simulink model "combinedTxRx_16bit"  (R2017a)
settings: Solver=FixedStepDiscrete  StartTime=0.0  StopTime=10.0  RelTol=1e-3
InitFcn:
  | numHeaderBits = 16;
  | %numPreambleBits = 250;
  | AGCBarkerSymbols = 160+28;
  | EQTrainingSymbols = 250;
  | CRCGeneratorLag = 34; % CRCLen + 2
  | 
  | %% AGC Preamble
  | B13bipolar = [0 0 0 0 0 2 2 0 0 2 0 2];
  | rep = [B13bipolar, B13bipolar(1:4)];
  | AGCBarker = repmat(rep,1,10);
  | % Second preamble part
  | B11bipolar = [0 0 0 2 2 2 0 2  2 0 2];
  | TimingBarker = [B11bipolar,B11bipolar,B11bipolar,B11bipolar(1:6)];
  | PreambleBarkersInts = [AGCBarker, TimingBarker];
  | % Convert integer into their bit representation
  | PreambleBarkersBits = zeros(1,length(PreambleBarkersInts)*2);
  | PreambleBarkersBits(1:2:end) = (PreambleBarkersInts==2);
  | 
  | % Constants
  | % First preamble part
  | B13bipolar = [0 0 0 0 0 2 2 0 0 2 0 2];
  | rep = [B13bipolar, B13bipolar(1:4)];
  | AGCBarker = repmat(rep,1,10);
  | % Second preamble part
  | B11bipolar = [0 0 0 2 2 2 0 2  2 0 2];
  | TimingBarker = [B11bipolar,B11bipolar,B11bipolar(1:6)];
  | PreambleBarkersInts = [AGCBarker, TimingBarker];
  | % Convert integer into their bit representation
  | PreambleBarkersBits = false(1,length(PreambleBarkersInts)*2);
  | PreambleBarkersBits(1:2:end) = logical(PreambleBarkersInts==2);
  | pLen = uint16(length(PreambleBarkersBits));
  | 
  | 
  | %%%%%%%%%%%%%%%%%%%%%%%%%%
  | %% RX
  | %%%%%%%%%%%%%%%%%%%%%%%%%%
  | 
  | barker = comm.BarkerCode('SamplesPerFrame', 28, 'Length', 11);
  | seq = barker()+1;
  | M = 4;
  | hPSKModTrain   = comm.PSKModulator(M, ...
  |     'PhaseOffset',pi/4, ...
  |     'SymbolMapping','Binary');
  | xPreambleSeq = hPSKModTrain(seq);
  | 
  | 
  | %%%%%%%%%%%%
  | 
  | % AGC Preamble
  | reps = 5;
  | barker = comm.BarkerCode('SamplesPerFrame', 16, 'Length', 13);
  | seq = barker()+1;
  | %preamble = zeros(16*reps,1);
  | preambleFull = repmat(seq,reps,1);
  | rctFilt = comm.RaisedCosineTransmitFilter('FilterSpanInSymbols', 128,...
  | 'RolloffFactor',0.5,...
  | 'OutputSamplesPerSymbol',4);
  | preambleFullFilt = rctFilt(preambleFull);
  | 
  | %%%%%%%%%%%%
  | 
  | RadioSampleRate = 1e6;
  | %RadioSampleRate = 20e6;
  | RadioFrameLength = 1e5;
  | 
  | VibertiTracebackLength = 34+20;
  | numTrainingSamples = 250;
  | crc32Poly = [1 0 0 0 0 0 1 0 0 1 1 0 0 0 0 0 1 0 0 0 1 1 1 0 1 1 0 1 1 0 1 1 1];
  | crcDecodeLag = length(crc32Poly)-1+2;
  | 
  | %%%%%%%%%%%%
  | 
  | beta = 0.5;
  | span = 8;
  | sps = 4;
  | filterGain = 1;
  | coeff = rcosdesign(beta, span, sps, 'sqrt')*filterGain;
  | 
  | %%%%%%%%%%%%
  | 
  | samplesPerSymbol = 4;
  | maxPacketBits = 8*1500;
  | bItsPerSymbol = 2;
  | CodeRate = 2;
  | tailSymbols = 40;
  | maxPayloadSymbols = maxPacketBits*CodeRate/bItsPerSymbol+tailSymbols;
undefined symbols (not defined in the file or in its folder): j
libraries: simulink x22, dsphdlfiltering x20, hdlsllib x6, commseqgen3 x4, dspsigops x4, commdigbbndpm3 x3, commcrc2 x2, commcnvcod2 x2, dspstat3 x2, commsource2 x1, commutil2 x1, commfilt2 x1
(part 1 of 3)
settings Model: Creator=tcollins  LastModifiedBy=tcollins
settings OptimizationCC: BlockReduction=off  ConditionallyExecuteInputs=off  DefaultParameterBehavior=Inlined
settings DebuggingCC: AlgebraicLoopMsg=error  SingleTaskRateTransMsg=error
settings HardwareCC: ProdBitPerPointer=32  ProdBitPerSizeT=32  ProdBitPerPtrDiffT=32  ProdLargestAtomicFloat=None  ProdIntDivRoundTo=Undefined  ProdEndianess=Unspecified  ProdWordSize=32  ProdHWDeviceType=ASIC/FPGA->ASIC/FPGA  ProdEqTarget=off

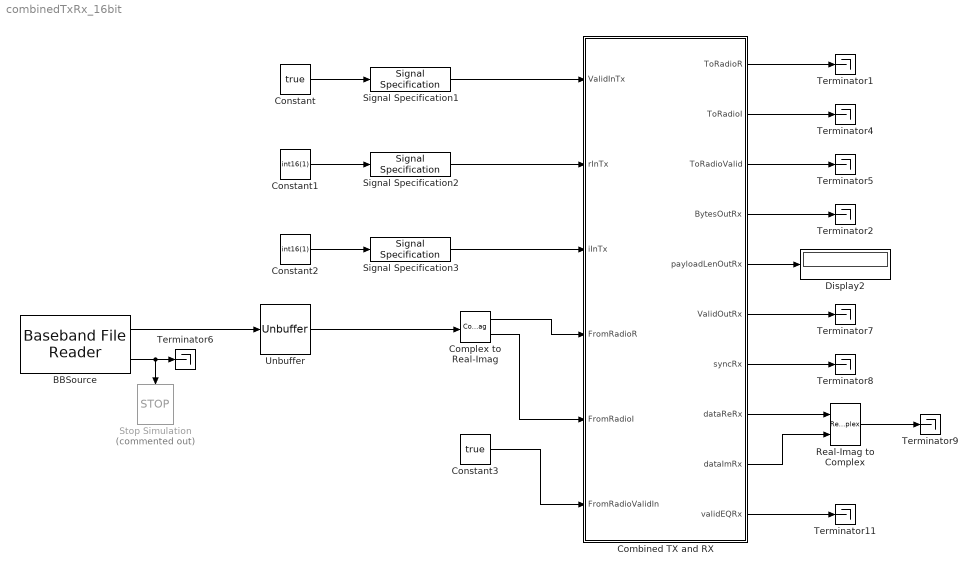
== system combinedTxRx_16bit ==
  BBSource : commsource2/Baseband File Reader  Filename=/home/tcollins/currentWork/modem-phy/FixedPoint/Pluto3.bb  InheritSampleTimeFromFile=off  SampleTime=100000/(RadioSampleRate)  SamplesPerFrame=100000  CyclicRepetition=off  FileEndOutputPort=on  SimulateUsing=Interpreted execution
      settings: SourceProductName=Communications System Toolbox  SourceProductBaseCode=CM
  Combined TX and RX : Subsystem  TreatAsAtomicUnit=on
  Complex to Real-Imag : ComplexToRealImag
  Constant : Constant  Value=true  SampleTime=-1
  Constant1 : Constant  Value=int16(1)  SampleTime=-1
  Constant2 : Constant  Value=int16(1)  SampleTime=-1
  Constant3 : Constant  Value=true  SampleTime=1/RadioSampleRate
  Display2 : Display
  Real-Imag to Complex : RealImagToComplex
  Signal Specification1 : SignalSpecification  OutDataTypeStr=boolean  SampleTime=1e-6
  Signal Specification2 : SignalSpecification  OutDataTypeStr=int16  SampleTime=1e-6
  Signal Specification3 : SignalSpecification  OutDataTypeStr=int16  SampleTime=1e-6
  Stop Simulation : Stop  Commented=on
  Terminator{1..2,4..9,11} (9 alike) : Terminator
  Unbuffer : Unbuffer
  wires:
  Constant1/1 -> Signal Specification2/1
  Constant2/1 -> Signal Specification3/1
  Constant/1 -> Signal Specification1/1
  Real-Imag to Complex/1 -> Terminator9/1
  BBSource/1 -> Unbuffer/1
  Unbuffer/1 -> Complex to Real-Imag/1
  BBSource/2 -> Stop Simulation/1, Terminator6/1
  Signal Specification1/1 -> Combined TX and RX/1(ValidInTx)
  Signal Specification2/1 -> Combined TX and RX/2(rInTx)
  Signal Specification3/1 -> Combined TX and RX/3(iInTx)
  Complex to Real-Imag/1 -> Combined TX and RX/4(FromRadioR)
  Complex to Real-Imag/2 -> Combined TX and RX/5(FromRadioI)
  Constant3/1 -> Combined TX and RX/6(FromRadioValidIn)
  Combined TX and RX/1(ToRadioR) -> Terminator1/1
  Combined TX and RX/2(ToRadioI) -> Terminator4/1
  Combined TX and RX/3(ToRadioValid) -> Terminator5/1
  Combined TX and RX/4(BytesOutRx) -> Terminator2/1
  Combined TX and RX/5(payloadLenOutRx) -> Display2/1
  Combined TX and RX/6(ValidOutRx) -> Terminator7/1
  Combined TX and RX/7(syncRx) -> Terminator8/1
  Combined TX and RX/8(dataReRx) -> Real-Imag to Complex/1
  Combined TX and RX/9(dataImRx) -> Real-Imag to Complex/2
  Combined TX and RX/10(validEQRx) -> Terminator11/1

== system combinedTxRx_16bit/Combined TX and RX ==
  ValidInTx : Inport
  rInTx : Inport  Port=2
  iInTx : Inport  Port=3
  FromRadioR : Inport  Port=4
  FromRadioI : Inport  Port=5
  FromRadioValidIn : Inport  Port=6
  Receiver HDL : Subsystem  TreatAsAtomicUnit=on
  Tx Under Test : Subsystem  TreatAsAtomicUnit=on
  ToRadioR : Outport
  ToRadioI : Outport  Port=2
  ToRadioValid : Outport  Port=3
  BytesOutRx : Outport  Port=4
  payloadLenOutRx : Outport  Port=5
  ValidOutRx : Outport  Port=6
  syncRx : Outport  Port=7
  dataReRx : Outport  Port=8
  dataImRx : Outport  Port=9
  validEQRx : Outport  Port=10
  wires:
  Receiver HDL/2(validOut) -> ValidOutRx/1
  Receiver HDL/6(dataIm) -> dataImRx/1
  Receiver HDL/3(sync) -> syncRx/1
  FromRadioI/1 -> Receiver HDL/2(Im)
  Receiver HDL/4(payloadLenOut) -> payloadLenOutRx/1
  Receiver HDL/7(validEQ) -> validEQRx/1
  Receiver HDL/5(dataRe) -> dataReRx/1
  FromRadioValidIn/1 -> Receiver HDL/3(Enable)
  FromRadioR/1 -> Receiver HDL/1(re)
  Receiver HDL/1(bytesOut) -> BytesOutRx/1
  rInTx/1 -> Tx Under Test/2("r ")
  Tx Under Test/2(Out2) -> ToRadioI/1
  Tx Under Test/3(Out3) -> ToRadioValid/1
  Tx Under Test/1(Out1) -> ToRadioR/1
  iInTx/1 -> Tx Under Test/3(i)
  ValidInTx/1 -> Tx Under Test/1(In1)

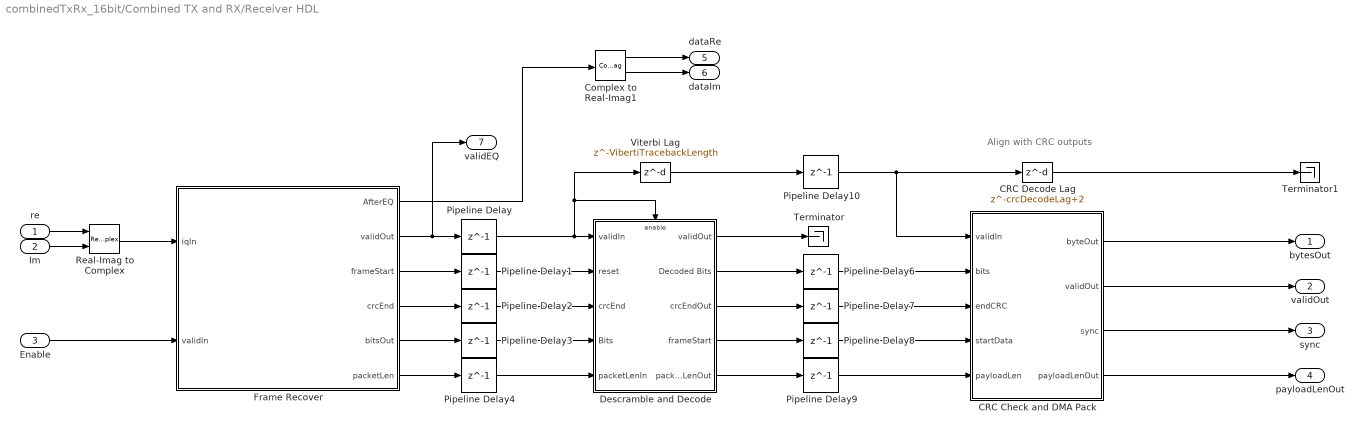
== system combinedTxRx_16bit/Combined TX and RX/Receiver HDL ==
  note: Align with CRC outputs
  re : Inport  OutDataTypeStr=int16
  Im : Inport  Port=2  OutDataTypeStr=int16
  Enable : Inport  Port=3
  CRC Check and DMA Pack : Subsystem
  CRC Decode Lag : Delay  DelayLength=crcDecodeLag+2
  Complex to Real-Imag1 : ComplexToRealImag
  Descramble and Decode : Subsystem  TreatAsAtomicUnit=on
  Frame Recover : Subsystem
  Pipeline Delay{,1..4,6..10} (10 alike) : Delay  DelayLength=1
  Real-Imag to Complex : RealImagToComplex
  Terminator : Terminator
  Terminator1 : Terminator
  Viterbi Lag : Delay  DelayLength=VibertiTracebackLength
  bytesOut : Outport
  validOut : Outport  Port=2
  sync : Outport  Port=3
  payloadLenOut : Outport  Port=4
  dataRe : Outport  Port=5
  dataIm : Outport  Port=6
  validEQ : Outport  Port=7
  wires:
  re/1 -> Real-Imag to Complex/1
  Im/1 -> Real-Imag to Complex/2
  Complex to Real-Imag1/2 -> dataIm/1
  Complex to Real-Imag1/1 -> dataRe/1
  Frame Recover/6(packetLen) -> Pipeline Delay4/1
  Frame Recover/2(validOut) -> validEQ/1, Pipeline Delay/1
  Real-Imag to Complex/1 -> Frame Recover/1(iqIn)
  Enable/1 -> Frame Recover/2(validIn)
  Frame Recover/1(AfterEQ) -> Complex to Real-Imag1/1
  Frame Recover/3(frameStart) -> Pipeline Delay1/1
  Frame Recover/4(crcEnd) -> Pipeline Delay2/1
  Frame Recover/5(bitsOut) -> Pipeline Delay3/1
  Descramble and Decode/3(crcEndOut) -> Pipeline Delay7/1
  Descramble and Decode/4(frameStart) -> Pipeline Delay8/1
  Descramble and Decode/5(packetLenOut) -> Pipeline Delay9/1
  CRC Check and DMA Pack/1(byteOut) -> bytesOut/1
  CRC Check and DMA Pack/2(validOut) -> validOut/1
  Pipeline Delay1/1 -> Descramble and Decode/2(reset)
  Pipeline Delay3/1 -> Descramble and Decode/4(Bits)
  Pipeline Delay4/1 -> Descramble and Decode/5(packetLenIn)
  Pipeline Delay8/1 -> CRC Check and DMA Pack/4(startData)
  Pipeline Delay6/1 -> CRC Check and DMA Pack/2(bits)
  Pipeline Delay9/1 -> CRC Check and DMA Pack/5(payloadLen)
  Pipeline Delay7/1 -> CRC Check and DMA Pack/3(endCRC)
  CRC Check and DMA Pack/3(sync) -> sync/1
  Pipeline Delay2/1 -> Descramble and Decode/3(crcEnd)
  Descramble and Decode/2(Decoded Bits) -> Pipeline Delay6/1
  Pipeline Delay10/1 -> CRC Check and DMA Pack/1(validIn), CRC Decode Lag/1
  CRC Check and DMA Pack/4(payloadLenOut) -> payloadLenOut/1
  Pipeline Delay/1 -> Descramble and Decode/Enable, Viterbi Lag/1, Descramble and Decode/1(validIn)
  Descramble and Decode/1(validOut) -> Terminator/1
  Viterbi Lag/1 -> Pipeline Delay10/1
  CRC Decode Lag/1 -> Terminator1/1

== system combinedTxRx_16bit/Combined TX and RX/Tx Under Test ==
  note: Keep On
  In1 : Inport
  "r " : Inport  Port=2
  i : Inport  Port=3
  DMA Model Driver : MATLAB Function  TreatAsAtomicUnit=on
  Data Type Conversion : DataTypeConversion  OutDataTypeStr=uint16
  Delay : Delay  DelayLength=1
  Downsample1 : DownSample  N=4  RateOptions=Allow multirate processing
  Downsample2 : DownSample  N=4  RateOptions=Allow multirate processing
  Logical Operator : Logic  Operator=OR  AllPortsSameDT=off  OutDataTypeStr=boolean
  Logical Operator1 : Logic  Operator=NOT  AllPortsSameDT=off  OutDataTypeStr=boolean
  Terminator : Terminator
  Terminator1 : Terminator
  Transmitter HDL : Subsystem  TreatAsAtomicUnit=on
  Upsample : dspsigops/Upsample  N=4  phase=0  RateOptions=Allow multirate processing  ic=0  mode=Unused parameter value
  Upsample1 : dspsigops/Upsample  N=4  phase=0  RateOptions=Allow multirate processing  ic=0  mode=Unused parameter value
  Out1 : Outport
  Out2 : Outport  Port=2
  Out3 : Outport  Port=3
  wires:
  Transmitter HDL/4(Need Data) -> Downsample1/1
  Transmitter HDL/2(imag) -> Out2/1
  Transmitter HDL/1(real) -> Out1/1
  Transmitter HDL/3(validOut) -> Out3/1
  DMA Model Driver/1(payload) -> Data Type Conversion/1
  Delay/1 -> DMA Model Driver/2(enable)
  In1/1 -> Downsample2/1
  Data Type Conversion/1 -> Upsample/1
  DMA Model Driver/2(valid) -> Upsample1/1
  "r "/1 -> Terminator/1
  i/1 -> Terminator1/1
  Upsample/1 -> Transmitter HDL/1(bytesIn)
  Upsample1/1 -> Transmitter HDL/2(validIn)
  Downsample1/1 -> Delay/1
  Logical Operator/1 -> DMA Model Driver/1(driver)
  Logical Operator1/1 -> Logical Operator/2
  Downsample2/1 -> Logical Operator1/1, Logical Operator/1

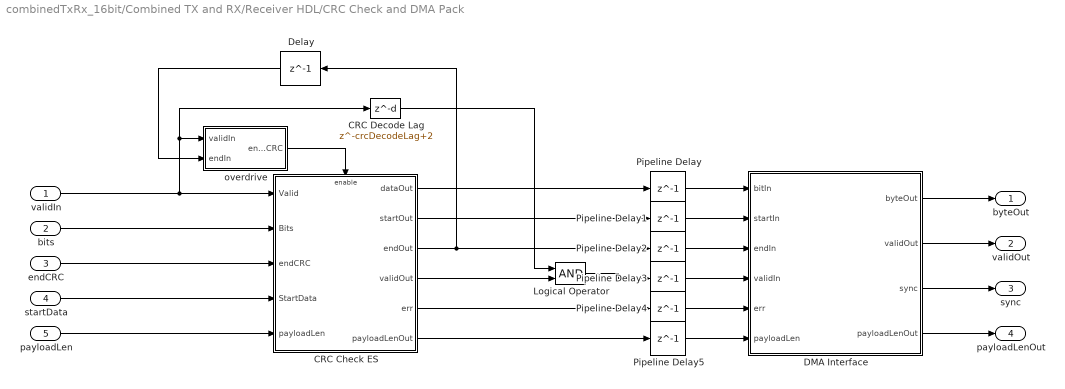
== system combinedTxRx_16bit/Combined TX and RX/Receiver HDL/CRC Check and DMA Pack ==
  validIn : Inport
  bits : Inport  Port=2
  endCRC : Inport  Port=3
  startData : Inport  Port=4
  payloadLen : Inport  Port=5
  CRC Check ES : Subsystem
  CRC Decode Lag : Delay  DelayLength=crcDecodeLag+2
  DMA Interface : Subsystem
  Delay : Delay  DelayLength=1
  Logical Operator : Logic  AllPortsSameDT=off  OutDataTypeStr=boolean
  Pipeline Delay{,1..5} (6 alike) : Delay  DelayLength=1
  overdrive : MATLAB Function  TreatAsAtomicUnit=on
  byteOut : Outport
  validOut : Outport  Port=2
  sync : Outport  Port=3
  payloadLenOut : Outport  Port=4
  wires:
  DMA Interface/2(validOut) -> validOut/1
  CRC Check ES/3(endOut) -> Delay/1, Pipeline Delay2/1
  DMA Interface/1(byteOut) -> byteOut/1
  CRC Check ES/2(startOut) -> Pipeline Delay1/1
  CRC Check ES/1(dataOut) -> Pipeline Delay/1
  CRC Check ES/5(err) -> Pipeline Delay4/1
  bits/1 -> CRC Check ES/2(Bits)
  DMA Interface/3(sync) -> sync/1
  payloadLen/1 -> CRC Check ES/5(payloadLen)
  startData/1 -> CRC Check ES/4(StartData)
  CRC Check ES/6(payloadLenOut) -> Pipeline Delay5/1
  endCRC/1 -> CRC Check ES/3(endCRC)
  Pipeline Delay/1 -> DMA Interface/1(bitIn)
  Pipeline Delay1/1 -> DMA Interface/2(startIn)
  Pipeline Delay2/1 -> DMA Interface/3(endIn)
  Pipeline Delay3/1 -> DMA Interface/4(validIn)
  Pipeline Delay4/1 -> DMA Interface/5(err)
  Pipeline Delay5/1 -> DMA Interface/6(payloadLen)
  CRC Decode Lag/1 -> Logical Operator/1
  CRC Check ES/4(validOut) -> Logical Operator/2
  validIn/1 -> CRC Check ES/1(Valid), CRC Decode Lag/1, overdrive/1(validIn)
  Delay/1 -> overdrive/2(endIn)
  DMA Interface/4(payloadLenOut) -> payloadLenOut/1
  Logical Operator/1 -> Pipeline Delay3/1
  overdrive/1(enableCRC) -> CRC Check ES/Enable

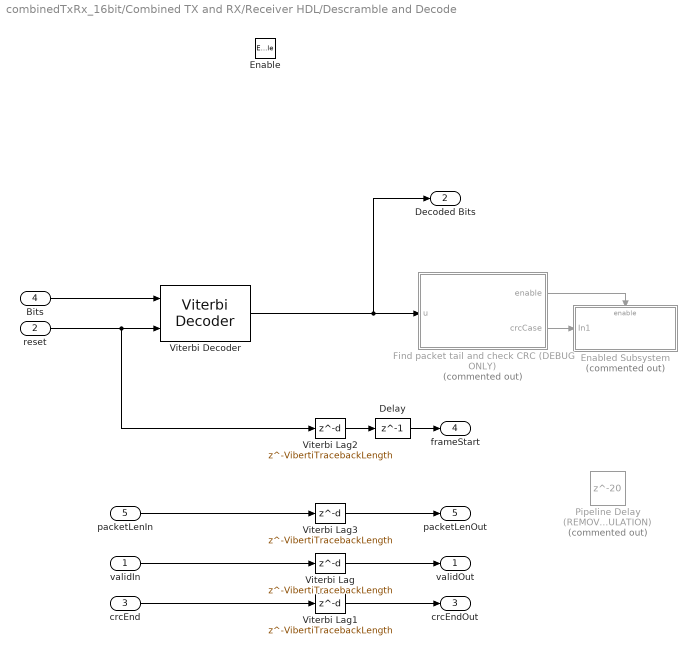
== system combinedTxRx_16bit/Combined TX and RX/Receiver HDL/Descramble and Decode ==
  validIn : Inport
  reset : Inport  Port=2
  crcEnd : Inport  Port=3
  Bits : Inport  Port=4
  packetLenIn : Inport  Port=5
  Enable : EnablePort
  Delay : Delay  DelayLength=1
  Enabled Subsystem : Subsystem  Commented=on  TreatAsAtomicUnit=on
  Find packet tail and check CRC (DEBUG ONLY) : MATLAB Function  Commented=on  TreatAsAtomicUnit=on
  "Pipeline Delay (REMOVE BEFORE SYNTH, ONLY FOR SIMULATION)" : Delay  Commented=on  DelayLength=20
  Viterbi Decoder : commcnvcod2/Viterbi Decoder  trellis=poly2trellis(7, [171 133])  isPunctured=off  punctureVector=[1; 1; 0; 1; 0; 1]  erasures=off  dectype=Hard decision  nsdecb=4  runSigValErrCheck=off  tbdepth=VibertiTracebackLength-20  opmode=Continuous  reset=on  delayedResetAction=on  smWordLength=16  outDataType=boolean
      settings: SourceProductName=Communications System Toolbox  SourceProductBaseCode=CM
  Viterbi Lag{,1..3} (4 alike) : Delay  DelayLength=VibertiTracebackLength
  validOut : Outport  InitialOutput=0
  Decoded Bits : Outport  Port=2  InitialOutput=0
  crcEndOut : Outport  Port=3  InitialOutput=0
  frameStart : Outport  Port=4  InitialOutput=0
  packetLenOut : Outport  Port=5  InitialOutput=0
  wires:
  reset/1 -> Viterbi Lag2/1, Viterbi Decoder/2
  Find packet tail and check CRC (DEBUG ONLY)/1(enable) -> Enabled Subsystem/Enable
  Find packet tail and check CRC (DEBUG ONLY)/2(crcCase) -> Enabled Subsystem/1(In1)
  Bits/1 -> Viterbi Decoder/1
  validIn/1 -> Viterbi Lag/1
  Viterbi Lag3/1 -> packetLenOut/1
  Viterbi Lag2/1 -> Delay/1
  Viterbi Lag1/1 -> crcEndOut/1
  Viterbi Lag/1 -> validOut/1
  packetLenIn/1 -> Viterbi Lag3/1
  crcEnd/1 -> Viterbi Lag1/1
  Delay/1 -> frameStart/1
  Viterbi Decoder/1 -> Decoded Bits/1, Find packet tail and check CRC (DEBUG ONLY)/1(u)

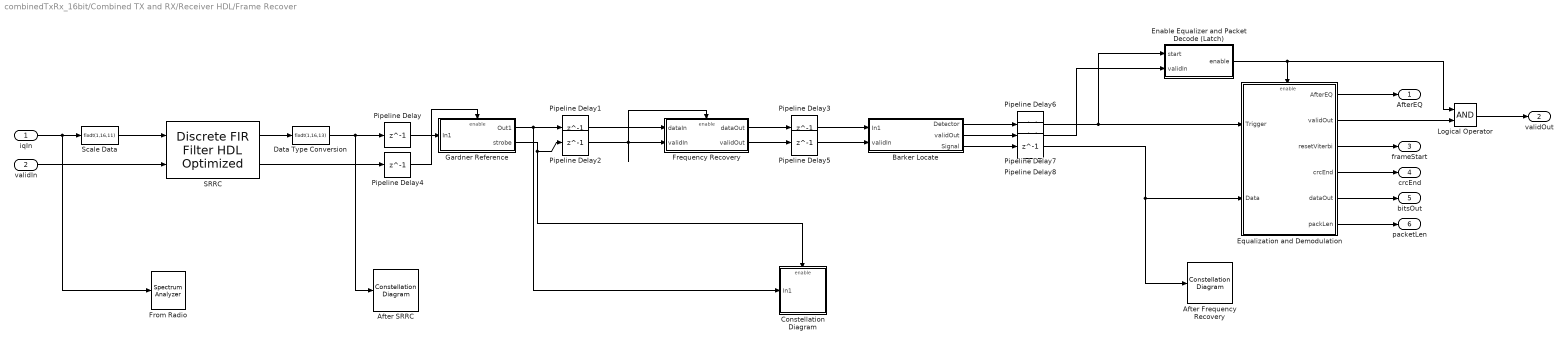
== system combinedTxRx_16bit/Combined TX and RX/Receiver HDL/Frame Recover ==
  iqIn : Inport
  validIn : Inport  Port=2
  After Frequency Recovery : ConstellationDiagram
  After SRRC : ConstellationDiagram
  Barker Locate : Subsystem  mask{Threshold=1}
  Constellation Diagram : Subsystem
  Data Type Conversion : DataTypeConversion  OutDataTypeStr=fixdt(1,16,13)
  Enable Equalizer and Packet Decode (Latch) : MATLAB Function  TreatAsAtomicUnit=on
  Equalization and Demodulation : Subsystem
  Frequency Recovery : Subsystem
  From Radio : SpectrumAnalyzer
  Gardner Reference : Subsystem
  Logical Operator : Logic  AllPortsSameDT=off  OutDataTypeStr=boolean
  Pipeline Delay{,1..8} (9 alike) : Delay  DelayLength=1
  SRRC : dsphdlfiltering/Discrete FIR Filter HDL Optimized  Numerator=coeff  Sharing=off  SharingFactor=2  SimulateUsing=Code generation  roundingMode=Floor  overflowMode=on  CoefficientsDataTypeStr=Inherit: Same word length as input  CoefficientsMin=[]  CoefficientsMax=[]  OutputDataTypeStr=fixdt(1,16,11)  OutputMin=[]  OutputMax=[]  ValidInPort=on  ReadyPort=off
      settings: SourceProductName=DSP System Toolbox  SourceProductBaseCode=DS
  Scale Data : DataTypeConversion  OutDataTypeStr=fixdt(1,16,11)  ConvertRealWorld=Stored Integer (SI)  SaturateOnIntegerOverflow=on
  AfterEQ : Outport
  validOut : Outport  Port=2
  frameStart : Outport  Port=3
  crcEnd : Outport  Port=4
  bitsOut : Outport  Port=5
  packetLen : Outport  Port=6
  wires:
  Equalization and Demodulation/3(resetViterbi) -> frameStart/1
  Barker Locate/2(validOut) -> Pipeline Delay7/1
  Equalization and Demodulation/4(crcEnd) -> crcEnd/1
  Frequency Recovery/2(validOut) -> Pipeline Delay5/1
  Enable Equalizer and Packet Decode (Latch)/1(enable) -> Logical Operator/1, Equalization and Demodulation/Enable
  Equalization and Demodulation/5(dataOut) -> bitsOut/1
  SRRC/2 -> Pipeline Delay4/1
  SRRC/1 -> Data Type Conversion/1
  iqIn/1 -> From Radio/1, Scale Data/1
  validIn/1 -> SRRC/2
  Barker Locate/3(Signal) -> Pipeline Delay8/1
  Frequency Recovery/1(dataOut) -> Pipeline Delay3/1
  Equalization and Demodulation/2(validOut) -> Logical Operator/2
  Scale Data/1 -> SRRC/1
  Equalization and Demodulation/6(packLen) -> packetLen/1
  Barker Locate/1(Detector) -> Pipeline Delay6/1
  Equalization and Demodulation/1(AfterEQ) -> AfterEQ/1
  Pipeline Delay1/1 -> Frequency Recovery/1(dataIn)
  Pipeline Delay2/1 -> Frequency Recovery/Enable, Frequency Recovery/2(validIn)
  Pipeline Delay3/1 -> Barker Locate/1(In1)
  Pipeline Delay5/1 -> Barker Locate/2(validIn)
  Pipeline Delay6/1 -> Enable Equalizer and Packet Decode (Latch)/1(start), Equalization and Demodulation/1(Trigger)
  Pipeline Delay7/1 -> Enable Equalizer and Packet Decode (Latch)/2(validIn)
  Pipeline Delay8/1 -> Equalization and Demodulation/2(Data), After Frequency Recovery/1
  Logical Operator/1 -> validOut/1
  Data Type Conversion/1 -> After SRRC/1, Pipeline Delay/1
  Pipeline Delay/1 -> Gardner Reference/1(In1)
  Gardner Reference/2(strobe) -> Pipeline Delay2/1, Constellation Diagram/Enable
  Gardner Reference/1(Out1) -> Constellation Diagram/1(In1), Pipeline Delay1/1
  Pipeline Delay4/1 -> Gardner Reference/Enable

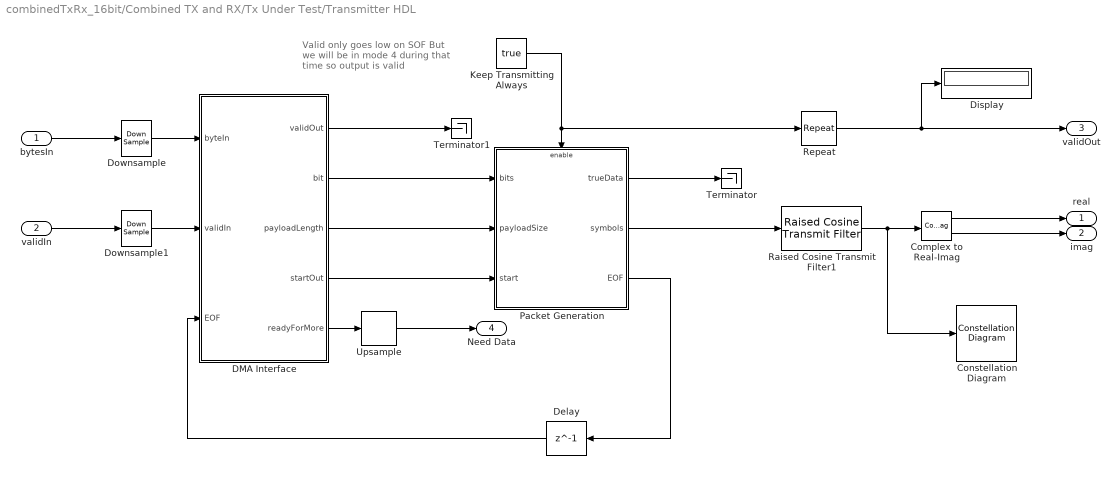
== system combinedTxRx_16bit/Combined TX and RX/Tx Under Test/Transmitter HDL ==
  note: Valid only goes low on SOF
      | But we will be in mode 4 during
      | that time so output is valid
  bytesIn : Inport
  validIn : Inport  Port=2
  Complex to Real-Imag : ComplexToRealImag
  Constellation Diagram : ConstellationDiagram
  DMA Interface : Subsystem
  Delay : Delay  DelayLength=1
  Display : Display
  Downsample : DownSample  N=4  RateOptions=Allow multirate processing
  Downsample1 : DownSample  N=4  RateOptions=Allow multirate processing
  Keep Transmitting Always : Constant  Value=true  SampleTime=-1
  Packet Generation : Subsystem
  Raised Cosine Transmit Filter1 : commfilt2/Raised Cosine Transmit Filter  filtType=Square root  R=0.5  filtSpan=8  N=4  filterGain=1  RateOptions=Allow multirate processing  framing=Mute  checkCoeff=off  variableName=rcTxFilt1  checkGain=Normalized  sampMode=Mute  saveAsFlag=0  currentFiltSpan=8  D=(8)/2  launchFVT=on  roundingMode=Floor  overflowMode=off  coeffDataTypeStr=Inherit: Same word length as input  coeffMin=[]  coeffMax=[]  coeffLastDataTypeStr=Inherit: Same word length as input  outputMode=Binary point scaling  outputWordLength=16  outputFracLength=14  outputDataTypeStr=fixdt(1,16,14)  outputMin=[]  outputMax=[]  outputLastDataTypeStr=fixdt(1,16,14)
  Repeat : dspsigops/Repeat  N=4  InputProcessing=Columns as channels (frame based)  RateOptions=Allow multirate processing  ic=0  mode=Unused parameter value
      settings: SourceProductName=DSP System Toolbox
  Terminator : Terminator
  Terminator1 : Terminator
  Upsample : dspsigops/Upsample  N=4  phase=0  RateOptions=Allow multirate processing  ic=0  mode=Unused parameter value
  real : Outport
  imag : Outport  Port=2
  validOut : Outport  Port=3
  Need Data : Outport  Port=4
  wires:
  Raised Cosine Transmit Filter1/1 -> Constellation Diagram/1, Complex to Real-Imag/1
  Complex to Real-Imag/1 -> real/1
  Complex to Real-Imag/2 -> imag/1
  DMA Interface/2(bit) -> Packet Generation/1(bits)
  DMA Interface/3(payloadLength) -> Packet Generation/2(payloadSize)
  DMA Interface/4(startOut) -> Packet Generation/3(start)
  Packet Generation/2(symbols) -> Raised Cosine Transmit Filter1/1
  DMA Interface/5(readyForMore) -> Upsample/1
  Repeat/1 -> validOut/1, Display/1
  Packet Generation/1(trueData) -> Terminator/1
  Packet Generation/3(EOF) -> Delay/1
  Delay/1 -> DMA Interface/3(EOF)
  bytesIn/1 -> Downsample/1
  validIn/1 -> Downsample1/1
  Upsample/1 -> Need Data/1
  Downsample/1 -> DMA Interface/1(byteIn)
  Downsample1/1 -> DMA Interface/2(validIn)
  DMA Interface/1(validOut) -> Terminator1/1
  Keep Transmitting Always/1 -> Packet Generation/Enable, Repeat/1

== system combinedTxRx_16bit/Combined TX and RX/Receiver HDL/CRC Check and DMA Pack/CRC Check ES ==
  note: NOTE:
      | 	The Valid signal must be latched during a packet, which is
      | 	a bug.  Therefore we must use the CRC block in an enabled
      | 	subsystem
  note: CRC Requires
      | Always High
      | Valid Signal During
      | Packet
  Valid : Inport
  Bits : Inport  Port=2
  endCRC : Inport  Port=3
  StartData : Inport  Port=4
  payloadLen : Inport  Port=5
  Enable : EnablePort
  CRC Decode Lag : Delay  DelayLength=crcDecodeLag
  Check CRC Result (DEBUG) : MATLAB Function  TreatAsAtomicUnit=on
  Convert To fi : DataTypeConversion  OutDataTypeStr=fixdt(0,1,0)  SaturateOnIntegerOverflow=on
  Debug CRC input : MATLAB Function  Commented=on  TreatAsAtomicUnit=on
  General CRC Syndrom Detector HDL Optimized : commcrc2/General CRC Syndrome Detector HDL Optimized  Polynomial=crc32Poly  InitialState=0  DirectMethod=off  ReflectInput=off  ReflectCRCChecksum=off  FinalXORValue=0  SimulateUsing=Code generation
      settings: SourceProductName=Communications System Toolbox  SourceProductBaseCode=CM
  dataOut : Outport  InitialOutput=0
  startOut : Outport  Port=2  InitialOutput=0
  endOut : Outport  Port=3  InitialOutput=0
  validOut : Outport  Port=4  InitialOutput=0
  err : Outport  Port=5  InitialOutput=0
  payloadLenOut : Outport  Port=6  InitialOutput=0
  wires:
  Bits/1 -> Convert To fi/1, Debug CRC input/1(u)
  General CRC Syndrom Detector HDL Optimized/1 -> Check CRC Result (DEBUG)/1(bits), dataOut/1
  General CRC Syndrom Detector HDL Optimized/3 -> Check CRC Result (DEBUG)/3(done), endOut/1
  General CRC Syndrom Detector HDL Optimized/4 -> Check CRC Result (DEBUG)/4(valid), validOut/1
  General CRC Syndrom Detector HDL Optimized/5 -> Check CRC Result (DEBUG)/5(err), err/1
  General CRC Syndrom Detector HDL Optimized/2 -> Check CRC Result (DEBUG)/2(start), startOut/1
  Convert To fi/1 -> General CRC Syndrom Detector HDL Optimized/1
  payloadLen/1 -> CRC Decode Lag/1
  CRC Decode Lag/1 -> payloadLenOut/1
  StartData/1 -> Debug CRC input/4(startFlag), General CRC Syndrom Detector HDL Optimized/2
  endCRC/1 -> Debug CRC input/3(endFlag), General CRC Syndrom Detector HDL Optimized/3
  Valid/1 -> Debug CRC input/2(enable), General CRC Syndrom Detector HDL Optimized/4

== system combinedTxRx_16bit/Combined TX and RX/Receiver HDL/CRC Check and DMA Pack/DMA Interface ==
  bitIn : Inport
  startIn : Inport  Port=2
  endIn : Inport  Port=3
  validIn : Inport  Port=4
  err : Inport  Port=5
  payloadLen : Inport  Port=6
  Bit Packer : MATLAB Function  TreatAsAtomicUnit=on
  Convert Payload Length To Bytes : Subsystem
  Data Type Conversion : DataTypeConversion  OutDataTypeStr=boolean
  Delay : Delay  DelayLength=1
  Delay Error To Last Byte of Out : Delay  DelayLength=1
  Display : Display
  byteOut : Outport
  validOut : Outport  Port=2
  sync : Outport  Port=3
  payloadLenOut : Outport  Port=4
  wires:
  bitIn/1 -> Data Type Conversion/1
  Delay/1 -> Bit Packer/3(endIn)
  Delay Error To Last Byte of Out/1 -> Bit Packer/4(err)
  Bit Packer/2(validOut) -> validOut/1
  Bit Packer/3(startOut) -> sync/1
  Bit Packer/1(byteOut) -> Display/1, byteOut/1
  err/1 -> Delay Error To Last Byte of Out/1
  validIn/1 -> Bit Packer/5(validIn)
  endIn/1 -> Delay/1
  startIn/1 -> Bit Packer/2(startIn)
  Data Type Conversion/1 -> Bit Packer/1(bitIn)
  payloadLen/1 -> Convert Payload Length To Bytes/1(In1)
  Convert Payload Length To Bytes/1(Out1) -> payloadLenOut/1

== system combinedTxRx_16bit/Combined TX and RX/Receiver HDL/Descramble and Decode/Enabled Subsystem ==
  In1 : Inport
  Enable : EnablePort
  To Workspace : ToWorkspace  VariableName=crcConditions  SaveFormat=Structure  SampleTime=-1
  wires:
  In1/1 -> To Workspace/1

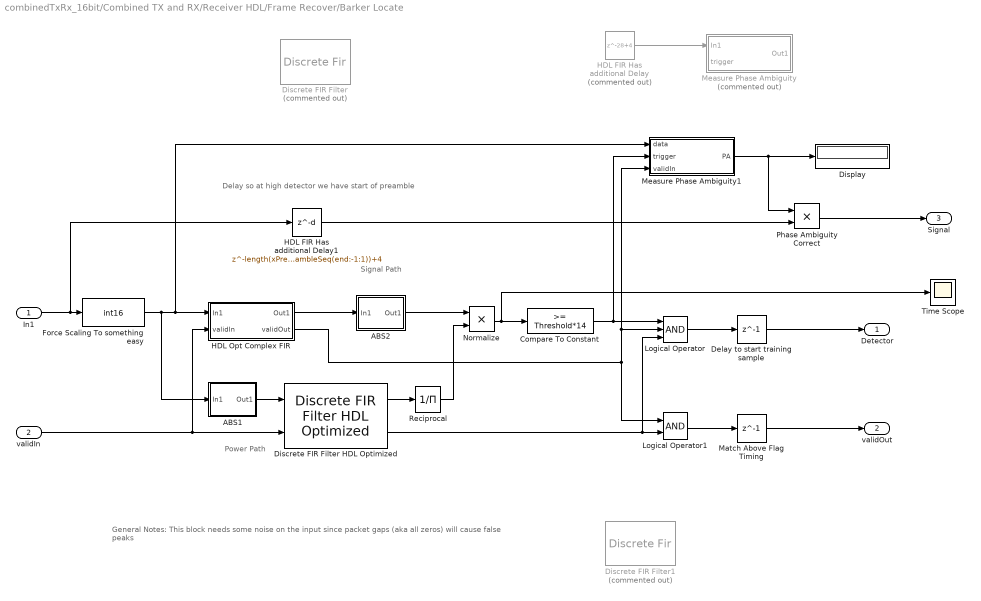
== system combinedTxRx_16bit/Combined TX and RX/Receiver HDL/Frame Recover/Barker Locate ==
  note: General Notes:
      | This block needs some noise on the input since packet gaps (aka all zeros) will cause false peaks
  note: Delay so at high detector we have start of preamble
  note: Power Path
  note: Signal Path
  In1 : Inport
  validIn : Inport  Port=2
  ABS1 : Subsystem
  ABS2 : Subsystem
  Compare To Constant : simulink/Logic and Bit Operations/Compare To Constant  relop=>=  const=Threshold*14  OutDataTypeStr=boolean
  "Delay to start training sample " : Delay  DelayLength=1
  Discrete FIR Filter : DiscreteFir  Commented=on  Coefficients=xPreambleSeq(end:-1:1).'  AccumDataTypeStr=Inherit: Same as product output  OutDataTypeStr=int16
  Discrete FIR Filter HDL Optimized : dsphdlfiltering/Discrete FIR Filter HDL Optimized  Numerator=ones(1,length(xPreambleSeq)*1)/1  Sharing=off  SharingFactor=2  SimulateUsing=Code generation  roundingMode=Floor  overflowMode=off  CoefficientsDataTypeStr=Inherit: Same word length as input  CoefficientsMin=[]  CoefficientsMax=[]  OutputDataTypeStr=fixdt(1,17,0)  OutputMin=[]  OutputMax=[]  ValidInPort=on  ReadyPort=off
      settings: SourceProductName=DSP System Toolbox  SourceProductBaseCode=DS
  Discrete FIR Filter1 : DiscreteFir  Commented=on  Coefficients=ones(1,length(xPreambleSeq)*1)/1  AccumDataTypeStr=Inherit: Same as product output  OutDataTypeStr=int16  SaturateOnIntegerOverflow=on
  Display : Display
  Force Scaling To something easy : DataTypeConversion  OutDataTypeStr=int16  SaturateOnIntegerOverflow=on
  HDL FIR Has additional Delay : Delay  Commented=on  DelayLength=28+4
  HDL FIR Has additional Delay1 : Delay  DelayLength=length(xPreambleSeq(end:-1:1))+4
  HDL Opt Complex FIR : Subsystem  mask{Taps=xPreambleSeq(end:-1:1).'}
  Logical Operator : Logic  Inputs=3  AllPortsSameDT=off  OutDataTypeStr=boolean
  Logical Operator1 : Logic  AllPortsSameDT=off  OutDataTypeStr=boolean
  Match Above Flag Timing : Delay  DelayLength=1
  Measure Phase Ambiguity : Subsystem  Commented=on
  Measure Phase Ambiguity1 : Subsystem
  Normalize : Product  Inputs=**  OutDataTypeStr=int16  RndMeth=Simplest  SaturateOnIntegerOverflow=on
  Phase Ambiguity Correct : Product  OutDataTypeStr=fixdt(1,16,14)
  Reciprocal : Product  Inputs=/  SaturateOnIntegerOverflow=on  RndMeth=Zero
  Time Scope : Scope
  Detector : Outport
  validOut : Outport  Port=2
  Signal : Outport  Port=3
  wires:
  HDL Opt Complex FIR/1(Out1) -> ABS2/1(In1)
  ABS2/1(Out1) -> Normalize/1
  "Delay to start training sample "/1 -> Detector/1
  Normalize/1 -> Time Scope/1, Compare To Constant/1
  In1/1 -> HDL FIR Has additional Delay1/1, Force Scaling To something easy/1
  ABS1/1(Out1) -> Discrete FIR Filter HDL Optimized/1
  Logical Operator/1 -> "Delay to start training sample "/1
  Logical Operator1/1 -> Match Above Flag Timing/1
  Measure Phase Ambiguity1/1(PA) -> Display/1, Phase Ambiguity Correct/1
  validIn/1 -> HDL Opt Complex FIR/2(validIn), Discrete FIR Filter HDL Optimized/2
  Discrete FIR Filter HDL Optimized/2 -> Logical Operator1/2, Logical Operator/3
  HDL Opt Complex FIR/2(validOut) -> Logical Operator1/1, Measure Phase Ambiguity1/3(validIn), Logical Operator/2
  Phase Ambiguity Correct/1 -> Signal/1
  HDL FIR Has additional Delay1/1 -> Phase Ambiguity Correct/2
  Force Scaling To something easy/1 -> ABS1/1(In1), HDL Opt Complex FIR/1(In1), Measure Phase Ambiguity1/1(data)
  Compare To Constant/1 -> Measure Phase Ambiguity1/2(trigger), Logical Operator/1
  HDL FIR Has additional Delay/1 -> Measure Phase Ambiguity/1(In1)
  Discrete FIR Filter HDL Optimized/1 -> Reciprocal/1
  Reciprocal/1 -> Normalize/2
  Match Above Flag Timing/1 -> validOut/1

== system combinedTxRx_16bit/Combined TX and RX/Receiver HDL/Frame Recover/Constellation Diagram ==
  In1 : Inport
  Enable : EnablePort
  After Timing Recovery : ConstellationDiagram
  wires:
  In1/1 -> After Timing Recovery/1

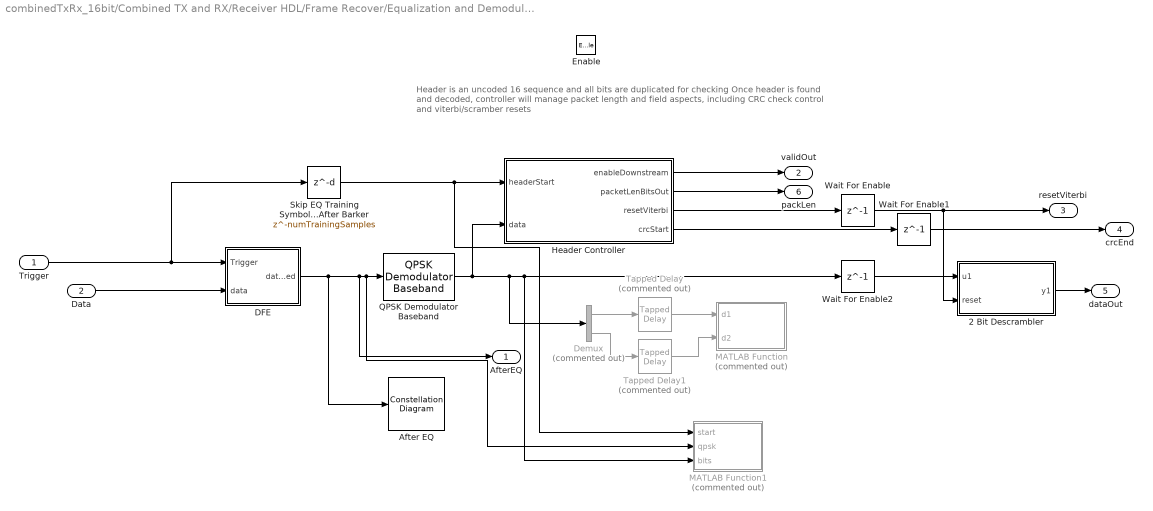
== system combinedTxRx_16bit/Combined TX and RX/Receiver HDL/Frame Recover/Equalization and Demodulation ==
  note: Header is an uncoded 16 sequence and all bits are duplicated for checking
      |
      | Once header is found and decoded, controller will manage packet length and field aspects,
      | including CRC check control and viterbi/scramber resets
  Trigger : Inport
  Data : Inport  Port=2
  Enable : EnablePort
  2 Bit Descrambler : Subsystem  mask{polynom=[1 1 0 1 0 1 0 1], initstate=[0 1 0 0 0 1 0]}
      mask prompts: polynom "Polynomial"; initstate "Inital State"
      mask Display: fprintf('HDL Descrambler')
  After EQ : ConstellationDiagram
  DFE : Subsystem
  Demux : Demux  Commented=on  Outputs=2
  Header Controller : MATLAB Function  TreatAsAtomicUnit=on
  MATLAB Function : MATLAB Function  Commented=on  TreatAsAtomicUnit=on
  MATLAB Function1 : MATLAB Function  Commented=on  TreatAsAtomicUnit=on
  QPSK Demodulator Baseband : commdigbbndpm3/QPSK Demodulator Baseband  OutType=Bit  DecType=Hard decision  VarSource=Dialog  Variance=1  Dec=Binary  Ph=pi/4  outDtype1=boolean  outDtype2=Inherit via internal rule  derotateFactorWordLen=16  derotateFactorDataTypeStr=Inherit: Same word length as input  derotateFactorLastDataTypeStr=Inherit: Same word length as input
  Skip EQ Training Symbols After Barker : Delay  DelayLength=numTrainingSamples
  Tapped Delay : simulink/Discrete/Tapped Delay  Commented=on  vinit=0.0  samptime=-1  NumDelays=16  DelayOrder=Oldest  includeCurrent=off
  Tapped Delay1 : simulink/Discrete/Tapped Delay  Commented=on  vinit=0.0  samptime=-1  NumDelays=16  DelayOrder=Oldest  includeCurrent=off
  Wait For Enable : Delay  DelayLength=1
  Wait For Enable1 : Delay  DelayLength=1
  Wait For Enable2 : Delay  DelayLength=1
  AfterEQ : Outport  InitialOutput=0
  validOut : Outport  Port=2  InitialOutput=0
  resetViterbi : Outport  Port=3  InitialOutput=0
  crcEnd : Outport  Port=4  InitialOutput=0
  dataOut : Outport  Port=5  InitialOutput=0
  packLen : Outport  Port=6  InitialOutput=0
  wires:
  Skip EQ Training Symbols After Barker/1 -> MATLAB Function1/1(start), Header Controller/1(headerStart)
  DFE/1(dataEQed) -> AfterEQ/1, MATLAB Function1/2(qpsk), QPSK Demodulator Baseband/1, After EQ/1
  QPSK Demodulator Baseband/1 -> Header Controller/2(data), Demux/1, MATLAB Function1/3(bits), Wait For Enable2/1
  Header Controller/1(enableDownstream) -> validOut/1
  Header Controller/4(crcStart) -> Wait For Enable1/1
  Header Controller/3(resetViterbi) -> Wait For Enable/1
  Header Controller/2(packetLenBitsOut) -> packLen/1
  Wait For Enable/1 -> 2 Bit Descrambler/2(reset), resetViterbi/1
  Wait For Enable1/1 -> crcEnd/1
  Wait For Enable2/1 -> 2 Bit Descrambler/1(u1)
  2 Bit Descrambler/1(y1) -> dataOut/1
  Demux/1 -> Tapped Delay/1
  Demux/2 -> Tapped Delay1/1
  Tapped Delay/1 -> MATLAB Function/1(d1)
  Tapped Delay1/1 -> MATLAB Function/2(d2)
  Trigger/1 -> DFE/1(Trigger), Skip EQ Training Symbols After Barker/1
  Data/1 -> DFE/2(data)

== system combinedTxRx_16bit/Combined TX and RX/Receiver HDL/Frame Recover/Frequency Recovery ==
  note: Decrease Loop bandwidth to reduce phase noise,
      | but worse pull-in range
      | -0.1 30kHz pull-in
      | -0.01 5kHz pull-in
  note: Max Phase Lock Delay= 1.3/(NormLoopBandwidth*SampleRate)
  note: Frequency Lock Delay = SampleRate*4*NormalizedPullInRange^2)/ (SampleRate*NormLoopBandwidth)^3;
  note: Pull in range (Hz) = 2*pi*sqrt(2)*DampingFactor*NormLoopBandwidth*SampleRate
  dataIn : Inport
  validIn : Inport  Port=2
  Enable : EnablePort
  Data Type Conversion : DataTypeConversion  Commented=on  OutDataTypeStr=fixdt(1,16,10)
  Delay : Delay  DelayLength=1
  Loop Filter : Subsystem  mask{BnTs=0.01, zeta=4*1/sqrt(2), N=1}
      mask prompts: BnTs "Normalized Loop Bandwidth"; zeta "Damping Factor"; N "Number of Samples/Symbol"
      mask init:
      | % See C.57 to C.61 in Michael Rice's "Digital Communications 
      | % - A Discrete-Time Approach" for details
      | 
      | %theta = BnTs/(zeta+0.25/zeta);  %0.0385
      | %d = 1 + 2*zeta*theta + theta*theta; %1.1938
      | %K1 = zeta*theta/d; %0.0805
      | %K2 = theta*theta/(d*2); %6.1958e-04
      | 
      | %%
      | DampingFactor = zeta;
      | samplesPerSymbol = N;
      | NormalizedLoopBandwidth = BnTs;
      | %
      | PhaseRecoveryLoopBandwidth = NormalizedLoopBandwidth*samplesPerSymbol;
      |  
      | PhaseRecoveryGain = samplesPerSymbol;
      |  
      | PhaseErrorDetectorGain = 1;
      | 
      | 
      | theta = PhaseRecoveryLoopBandwidth/...
      |     ((DampingFactor + 0.25/DampingFactor)*samplesPerSymbol);
      |  
      | d = 1 + 2*DampingFactor*theta + theta*theta;
      |  
      | % K1
      | K1 = (4*DampingFactor*theta/d)/...
      |     (PhaseErrorDetectorGain*PhaseRecoveryGain);
      | % K2
      | K2 = (4/samplesPerSymbol*theta*theta/d)/...
      |     (PhaseErrorDetectorGain*PhaseRecoveryGain);
      mask Display: disp('Loop Filter')
  PED : MATLAB Function  TreatAsAtomicUnit=on
  PED For QPSK : Subsystem  Commented=on
  PED For QPSK1 : Subsystem  Commented=on
  Phase Shift FP : Subsystem
  State Control : StateControl  StateControl=Synchronous
  dataOut : Outport
  validOut : Outport  Port=2
  wires:
  Delay/1 -> PED/1(In), dataOut/1
  PED/1(e) -> Loop Filter/1(e)
  Loop Filter/1(v) -> Phase Shift FP/2(Phi)
  dataIn/1 -> Phase Shift FP/1(In1)
  Phase Shift FP/1(Out1) -> Delay/1
  validIn/1 -> validOut/1

== system combinedTxRx_16bit/Combined TX and RX/Receiver HDL/Frame Recover/Gardner Reference ==
  In1 : Inport
  Enable : EnablePort
  Delay : Delay  DelayLength=1
  Delay1 : Delay  DelayLength=1
  Delay2 : Delay  DelayLength=6
  Gardner TED Blocks : Subsystem
  InterpControl_Blocks1 : Subsystem
  Interpolator : Subsystem
  LoopFilter1 : Subsystem  mask{zeta=sqrt(2), BnTs=0.01, Kp=2.7}
      mask prompts: zeta "DampingFactor"; BnTs "NormalizedLoopBandwidth"; Kp "DetectionGain"
      mask init:
      | K0 = -1;
      | SPS = 4;
      | theta = BnTs/SPS/(zeta + 0.25/zeta);
      | d  = (1 + 2*zeta*theta + theta^2) * K0 * Kp;
      | ProportionalGain = (4*zeta*theta) /d;
      | IntegratorGain   = (4*theta*theta)/d;
  State Control : StateControl  StateControl=Synchronous
  Out1 : Outport  InitialOutput=0
  strobe : Outport  Port=2  InitialOutput=false
  wires:
  In1/1 -> Delay2/1
  Delay1/1 -> Gardner TED Blocks/2(strobe), strobe/1
  Delay/1 -> Interpolator/2(mu)
  Interpolator/1(Out1) -> Gardner TED Blocks/1(data), Out1/1
  Gardner TED Blocks/1(e) -> LoopFilter1/1(e)
  InterpControl_Blocks1/1(strobe) -> Delay1/1
  InterpControl_Blocks1/2(mu) -> Delay/1
  LoopFilter1/1(v) -> InterpControl_Blocks1/1(e)
  Delay2/1 -> Interpolator/1(In1)

== system combinedTxRx_16bit/Combined TX and RX/Tx Under Test/Transmitter HDL/DMA Interface ==
  byteIn : Inport
  validIn : Inport  Port=2
  EOF : Inport  Port=3
  Align with data : Delay  DelayLength=1
  DMA Control : MATLAB Function  TreatAsAtomicUnit=on
  validOut : Outport
  bit : Outport  Port=2
  payloadLength : Outport  Port=3  OutDataTypeStr=uint16
  startOut : Outport  Port=4
  readyForMore : Outport  Port=5
  wires:
  byteIn/1 -> DMA Control/1(byteIn)
  DMA Control/1(bitOut) -> bit/1
  DMA Control/5(readyForInput) -> readyForMore/1
  DMA Control/4(payloadLength) -> payloadLength/1
  DMA Control/2(validOut) -> validOut/1
  validIn/1 -> DMA Control/2(validIn)
  Align with data/1 -> startOut/1
  DMA Control/3(startOut) -> Align with data/1
  EOF/1 -> DMA Control/3(EOF)

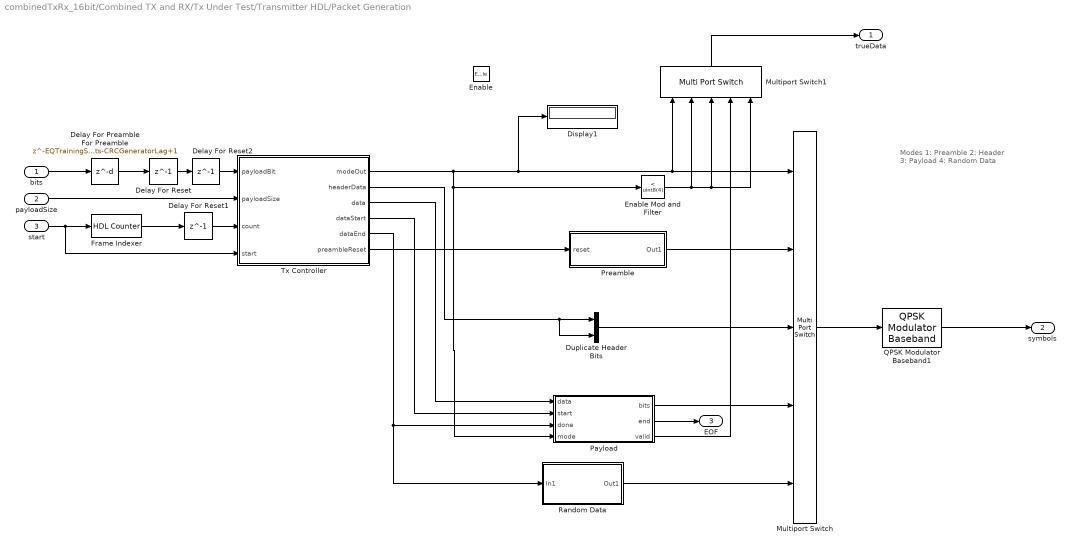
== system combinedTxRx_16bit/Combined TX and RX/Tx Under Test/Transmitter HDL/Packet Generation ==
  note: Modes
      | 	1: Preamble
      | 	2: Header
      | 	3: Payload
      | 	4: Random Data
  bits : Inport  OutDataTypeStr=boolean
  payloadSize : Inport  Port=2
  start : Inport  Port=3
  Enable : EnablePort
  Delay For Preamble For Preamble : Delay  DelayLength=EQTrainingSymbols+AGCBarkerSymbols+numHeaderBits-CRCGeneratorLag+1  InitialCondition=false
  Delay For Reset : Delay  DelayLength=1  InitialCondition=false
  Delay For Reset1 : Delay  DelayLength=1
  Delay For Reset2 : Delay  DelayLength=1  InitialCondition=false
  Display1 : Display
  Duplicate Header Bits : Concatenate
  Enable Mod and Filter : simulink/Logic and Bit Operations/Compare To Constant  relop=<  const=uint8(4)  OutDataTypeStr=boolean
  Frame Indexer : hdlsllib/HDL Operations/HDL Counter  CountType=Count limited  CountInit=0  CountStep=1  CountMax=2^16+EQTrainingSymbols+AGCBarkerSymbols+numHeaderBits  CountFromType=Specify  CountFrom=0  CountResetPort=on  CountLoadPort=off  CountEnbPort=off  CountDirPort=off  CountDataType=Unsigned  CountWordLen=32  CountFracLen=0  CountSampTime=1
      settings: SourceProductName=HDL Coder  SourceProductBaseCode=HD
  Multiport Switch : MultiPortSwitch  Inputs=4
  Multiport Switch1 : MultiPortSwitch  Inputs=4
  Payload : Subsystem
  Preamble : Subsystem
  QPSK Modulator Baseband1 : commdigbbndpm3/QPSK Modulator Baseband  InType=Bit  Enc=Binary  Ph=pi/4  outDtype=Fixed-point  outWordLen=16  outUDDataType=sfix(16)  outFracLenMode=User-defined  outFracLen=15  outDataTypeStr=fixdt(1,16,15)  outLastDataTypeStr=fixdt(1,16,15)
  Random Data : Subsystem
  Tx Controller : MATLAB Function  TreatAsAtomicUnit=on
  trueData : Outport  InitialOutput=0
  symbols : Outport  Port=2  InitialOutput=complex(0)
  EOF : Outport  Port=3  OutDataTypeStr=boolean  InitialOutput=0
  wires:
  Tx Controller/2(headerData) -> Duplicate Header Bits/2, Duplicate Header Bits/1
  Random Data/1(Out1) -> Multiport Switch/5
  Enable Mod and Filter/1 -> Multiport Switch1/5, Multiport Switch1/3, Multiport Switch1/2
  Tx Controller/3(data) -> Payload/1(data)
  Tx Controller/4(dataStart) -> Payload/2(start)
  Delay For Reset/1 -> Delay For Reset2/1
  start/1 -> Tx Controller/4(start), Frame Indexer/1
  Preamble/1(Out1) -> Multiport Switch/2
  bits/1 -> Delay For Preamble For Preamble/1
  QPSK Modulator Baseband1/1 -> symbols/1
  Multiport Switch1/1 -> trueData/1
  Delay For Reset1/1 -> Tx Controller/3(count)
  Multiport Switch/1 -> QPSK Modulator Baseband1/1
  Tx Controller/5(dataEnd) -> Payload/3(done), Random Data/1(In1)
  Payload/1(bits) -> Multiport Switch/4
  Duplicate Header Bits/1 -> Multiport Switch/3
  Frame Indexer/1 -> Delay For Reset1/1
  Payload/3(valid) -> Multiport Switch1/4
  Payload/2(end) -> EOF/1
  payloadSize/1 -> Tx Controller/2(payloadSize)
  Delay For Preamble For Preamble/1 -> Delay For Reset/1
  Tx Controller/1(modeOut) -> Display1/1, Multiport Switch/1, Multiport Switch1/1, Payload/4(mode), Enable Mod and Filter/1
  Tx Controller/6(preambleReset) -> Preamble/1(reset)
  Delay For Reset2/1 -> Tx Controller/1(payloadBit)

== system combinedTxRx_16bit/Combined TX and RX/Receiver HDL/CRC Check and DMA Pack/DMA Interface/Convert Payload Length To Bytes ==
  In1 : Inport
  Constant : Constant  Value=uint16(32-1)  SampleTime=-1
  Convert To Bytes From Bits : ArithShift  BitShiftNumber=3  BitShiftDirection=Right
  Convert To Uncoded : ArithShift  BitShiftNumber=1  BitShiftDirection=Right
  Data Type Conversion : DataTypeConversion  OutDataTypeStr=uint16
  Remove CRC Length : Sum  Inputs=+-  AccumDataTypeStr=uint16
  Out1 : Outport
  wires:
  In1/1 -> Convert To Uncoded/1
  Remove CRC Length/1 -> Convert To Bytes From Bits/1
  Convert To Uncoded/1 -> Remove CRC Length/1
  Convert To Bytes From Bits/1 -> Data Type Conversion/1
  Constant/1 -> Remove CRC Length/2
  Data Type Conversion/1 -> Out1/1

== system combinedTxRx_16bit/Combined TX and RX/Receiver HDL/Frame Recover/Barker Locate/ABS1 ==
  In1 : Inport
  Add : Sum
  Complex to Real-Imag : ComplexToRealImag
  Product : Product  OutDataTypeStr=int16
  Product1 : Product  OutDataTypeStr=int16
  Out1 : Outport
  wires:
  In1/1 -> Complex to Real-Imag/1
  Complex to Real-Imag/2 -> Product1/2, Product1/1
  Complex to Real-Imag/1 -> Product/1, Product/2
  Product/1 -> Add/1
  Product1/1 -> Add/2
  Add/1 -> Out1/1

== system combinedTxRx_16bit/Combined TX and RX/Receiver HDL/Frame Recover/Barker Locate/ABS2 ==
  In1 : Inport
  Add : Sum  SaturateOnIntegerOverflow=on
  Complex to Real-Imag : ComplexToRealImag
  Product : Product  OutDataTypeStr=int16
  Product1 : Product  OutDataTypeStr=int16
  Out1 : Outport
  wires:
  In1/1 -> Complex to Real-Imag/1
  Complex to Real-Imag/2 -> Product1/2, Product1/1
  Complex to Real-Imag/1 -> Product/1, Product/2
  Product/1 -> Add/1
  Product1/1 -> Add/2
  Add/1 -> Out1/1

== system combinedTxRx_16bit/Combined TX and RX/Receiver HDL/Frame Recover/Barker Locate/HDL Opt Complex FIR ==
  In1 : Inport
  validIn : Inport  Port=2
  Add : Sum  AccumDataTypeStr=fixdt(1,16,0)
  Discrete FIR Filter HDL Optimized : dsphdlfiltering/Discrete FIR Filter HDL Optimized  Numerator=real(Taps)  Sharing=off  SharingFactor=2  SimulateUsing=Code generation  roundingMode=Floor  overflowMode=off  CoefficientsDataTypeStr=Inherit: Same word length as input  CoefficientsMin=[]  CoefficientsMax=[]  OutputDataTypeStr=fixdt(1,15,0)  OutputMin=[]  OutputMax=[]  ValidInPort=on  ReadyPort=off
      settings: SourceProductName=DSP System Toolbox  SourceProductBaseCode=DS
  Discrete FIR Filter HDL Optimized1 : dsphdlfiltering/Discrete FIR Filter HDL Optimized  Numerator=imag(Taps)  Sharing=off  SharingFactor=2  SimulateUsing=Code generation  roundingMode=Floor  overflowMode=off  CoefficientsDataTypeStr=Inherit: Same word length as input  CoefficientsMin=[]  CoefficientsMax=[]  OutputDataTypeStr=fixdt(1,15,0)  OutputMin=[]  OutputMax=[]  ValidInPort=on  ReadyPort=off
      settings: SourceProductName=DSP System Toolbox  SourceProductBaseCode=DS
  Logical Operator : Logic  AllPortsSameDT=off  OutDataTypeStr=boolean
  Out1 : Outport
  validOut : Outport  Port=2
  wires:
  In1/1 -> Discrete FIR Filter HDL Optimized1/1, Discrete FIR Filter HDL Optimized/1
  Discrete FIR Filter HDL Optimized/1 -> Add/1
  Add/1 -> Out1/1
  Logical Operator/1 -> validOut/1
  Discrete FIR Filter HDL Optimized/2 -> Logical Operator/1
  Discrete FIR Filter HDL Optimized1/2 -> Logical Operator/2
  Discrete FIR Filter HDL Optimized1/1 -> Add/2
  validIn/1 -> Discrete FIR Filter HDL Optimized1/2, Discrete FIR Filter HDL Optimized/2

== system combinedTxRx_16bit/Combined TX and RX/Receiver HDL/Frame Recover/Barker Locate/Measure Phase Ambiguity ==
  In1 : Inport  OutDataTypeStr=int16
  trigger : Inport  Port=2
  Discrete FIR Filter1 : DiscreteFir  Coefficients=exp(-j*pi/2).*xPreambleSeq(end:-1:1).'  AccumDataTypeStr=Inherit: Same as product output  OutDataTypeStr=int16
  Discrete FIR Filter2 : DiscreteFir  Coefficients=xPreambleSeq(end:-1:1).'  AccumDataTypeStr=Inherit: Same as product output  OutDataTypeStr=int16
  Discrete FIR Filter3 : DiscreteFir  Coefficients=exp(-j*pi).*xPreambleSeq(end:-1:1).'  AccumDataTypeStr=Inherit: Same as product output  OutDataTypeStr=int16
  Discrete FIR Filter4 : DiscreteFir  Coefficients=exp(-j*pi*3/2).*xPreambleSeq(end:-1:1).'  AccumDataTypeStr=Inherit: Same as product output  OutDataTypeStr=int16
  Find Max and Set Output Shift : Subsystem
  Out1 : Outport  InitialOutput=0
  wires:
  In1/1 -> Discrete FIR Filter4/1, Discrete FIR Filter3/1, Discrete FIR Filter1/1, Discrete FIR Filter2/1
  Discrete FIR Filter2/1 -> Find Max and Set Output Shift/1(In1)
  Discrete FIR Filter1/1 -> Find Max and Set Output Shift/2(In2)
  Discrete FIR Filter3/1 -> Find Max and Set Output Shift/3(In4)
  Discrete FIR Filter4/1 -> Find Max and Set Output Shift/4(In5)
  trigger/1 -> Find Max and Set Output Shift/Enable
  Find Max and Set Output Shift/1(Out1) -> Out1/1

== system combinedTxRx_16bit/Combined TX and RX/Receiver HDL/Frame Recover/Barker Locate/Measure Phase Ambiguity1 ==
  data : Inport  OutDataTypeStr=int16
  trigger : Inport  Port=2
  validIn : Inport  Port=3
  Find Max and Set Output Shift : Subsystem
  HDL Opt Complex FIR4 : Subsystem  mask{Taps=xPreambleSeq(end:-1:1).'}
  HDL Opt Complex FIR5 : Subsystem  mask{Taps=exp(-j*pi/2).*xPreambleSeq(end:-1:1).'}
  HDL Opt Complex FIR6 : Subsystem  mask{Taps=exp(-j*pi).*xPreambleSeq(end:-1:1).'}
  HDL Opt Complex FIR7 : Subsystem  mask{Taps=exp(-j*pi*3/2).*xPreambleSeq(end:-1:1).'}
  Logical Operator : Logic  Inputs=5  AllPortsSameDT=off  OutDataTypeStr=boolean
  PA : Outport  InitialOutput=0
  wires:
  data/1 -> HDL Opt Complex FIR4/1(In1), HDL Opt Complex FIR5/1(In1), HDL Opt Complex FIR7/1(In1), HDL Opt Complex FIR6/1(In1)
  HDL Opt Complex FIR4/1(Out1) -> Find Max and Set Output Shift/1(In1)
  HDL Opt Complex FIR5/1(Out1) -> Find Max and Set Output Shift/2(In2)
  HDL Opt Complex FIR6/1(Out1) -> Find Max and Set Output Shift/3(In4)
  HDL Opt Complex FIR7/1(Out1) -> Find Max and Set Output Shift/4(In5)
  Find Max and Set Output Shift/1(Out1) -> PA/1
  validIn/1 -> HDL Opt Complex FIR4/2(validIn), HDL Opt Complex FIR5/2(validIn), HDL Opt Complex FIR7/2(validIn), HDL Opt Complex FIR6/2(validIn)
  HDL Opt Complex FIR4/2(validOut) -> Logical Operator/1
  HDL Opt Complex FIR5/2(validOut) -> Logical Operator/2
  HDL Opt Complex FIR6/2(validOut) -> Logical Operator/3
  HDL Opt Complex FIR7/2(validOut) -> Logical Operator/4
  Logical Operator/1 -> Find Max and Set Output Shift/Enable
  trigger/1 -> Logical Operator/5

== system combinedTxRx_16bit/Combined TX and RX/Receiver HDL/Frame Recover/Equalization and Demodulation/2 Bit Descrambler ==
  note: This is a special Descrambler which can process 2 bits at a time
  u1 : Inport
  reset : Inport  Port=2
  Demux1 : Demux  Outputs=2
  MATLAB Function : MATLAB Function  TreatAsAtomicUnit=on
  Mux : Mux  Inputs=2
  Selector1 : Selector  IndexOptions=Index vector (dialog)  Indices=find(polynom(2:end))  OutputSizes=1
  Selector2 : Selector  IndexOptions=Index vector (dialog)  Indices=find(polynom(2:end))  OutputSizes=1
  input_xor1 : Logic  Operator=XOR  IconShape=distinctive  AllPortsSameDT=off  OutDataTypeStr=boolean
  input_xor2 : Logic  Operator=XOR  IconShape=distinctive  AllPortsSameDT=off  OutDataTypeStr=boolean
  state_xor1 : Logic  Operator=XOR  Inputs=1  IconShape=distinctive  AllPortsSameDT=off  OutDataTypeStr=boolean
  state_xor2 : Logic  Operator=XOR  Inputs=1  IconShape=distinctive  AllPortsSameDT=off  OutDataTypeStr=boolean
  y1 : Outport  InitialOutput=0
  wires:
  u1/1 -> Demux1/1, MATLAB Function/1(bits)
  reset/1 -> MATLAB Function/2(reset)
  MATLAB Function/1(bufferA) -> Selector1/1
  MATLAB Function/2(bufferB) -> Selector2/1
  Mux/1 -> y1/1
  state_xor1/1 -> input_xor1/1
  state_xor2/1 -> input_xor2/1
  input_xor2/1 -> Mux/2
  input_xor1/1 -> Mux/1
  Selector1/1 -> state_xor1/1
  Selector2/1 -> state_xor2/1
  Demux1/1 -> input_xor1/2
  Demux1/2 -> input_xor2/2  "data_in"

== system combinedTxRx_16bit/Combined TX and RX/Receiver HDL/Frame Recover/Equalization and Demodulation/DFE ==
  note: Generate training sequence when barker is found
  Trigger : Inport
  data : Inport  Port=2
  Delay data so DFE can reset : Delay  DelayLength=1
  Delay ref so DFE can reset : Delay  DelayLength=1
  Equalizer : MATLAB Function  TreatAsAtomicUnit=on
  PN Sequence Generator : commseqgen3/PN Sequence Generator  poly='z^5 + z^3 + z^1 + 1'  ini_sta=[1 1 1 0 0]  outBitMaskSource=Dialog parameter  shift=0  outVarSiz=off  maxOutSizeMode=Dialog parameter  maxOutSize=[10 1]  Ts=-1  sampPerFrame=1  reset=on  bitPackedOutputs=on  outDataType=Smallest unsigned integer  numPackedBits=2  bitPackDataSigned=off  bitPackedOutDType=Smallest integer
      settings: SourceProductName=Communications System Toolbox
  Packeted To Unpacked : Subsystem
  QPSK Modulator Baseband : commdigbbndpm3/QPSK Modulator Baseband  InType=Bit  Enc=Binary  Ph=pi/4  outDtype=Fixed-point  outWordLen=16  outUDDataType=sfix(16)  outFracLenMode=User-defined  outFracLen=14  outDataTypeStr=fixdt(1,16,14)  outLastDataTypeStr=fixdt(1,16,14)
  dataEQed : Outport
  wires:
  Trigger/1 -> Equalizer/1(trigger), PN Sequence Generator/1
  data/1 -> Delay data so DFE can reset/1
  PN Sequence Generator/1 -> Packeted To Unpacked/1(In1)
  Packeted To Unpacked/1(Out1) -> QPSK Modulator Baseband/1
  QPSK Modulator Baseband/1 -> Delay ref so DFE can reset/1
  Delay data so DFE can reset/1 -> Equalizer/2(data)
  Delay ref so DFE can reset/1 -> Equalizer/3(trainingSymbol)
  Equalizer/1(eqOut) -> dataEQed/1

== system combinedTxRx_16bit/Combined TX and RX/Receiver HDL/Frame Recover/Frequency Recovery/Loop Filter ==
  note: This inflation is necessary
  note: Proportional-plus-Integrator Loop Filter,
      | Infinite DC Response to guarantee convergence
  e : Inport
  Add1 : Sum  RndMeth=Nearest  OutDataTypeStr=Inherit: Same as first input
  Add2 : Sum  OutDataTypeStr=Inherit: Same as first input
  Data Type Conversion : DataTypeConversion  OutDataTypeStr=fixdt(1,25,20)
  Delay : Delay  DelayLength=1
  Delay3 : Delay  DelayLength=1
  Delay4 : Delay  DelayLength=1
  Flip Sign : MATLAB Function  Commented=on  TreatAsAtomicUnit=on
  Gain : Gain  Commented=on  Gain=-1.0  OutDataTypeStr=fixdt(1,25,20)
  K1 : Gain  Gain=K2  OutDataTypeStr=Inherit: Same as input
  K2 : Gain  Gain=K1  OutDataTypeStr=Inherit: Same as input
  Sum2 : Sum  OutDataTypeStr=Inherit: Same as first input
  v : Outport
  wires:
  K1/1 -> Sum2/1
  Add1/1 -> Sum2/2
  e/1 -> K2/1, K1/1
  K2/1 -> Delay/1, Add1/2
  Delay/1 -> Add1/1
  Sum2/1 -> Delay3/1
  Delay3/1 -> Add2/1
  Delay4/1 -> Add2/2
  Add2/1 -> Delay4/1, Flip Sign/1(u), Data Type Conversion/1, Gain/1
  Data Type Conversion/1 -> v/1
